simulink model "vehicle_model10DOF_2023b"  (R2023b)
settings: Solver=VariableStepAuto  StartTime=0.0  StopTime=10.0  RelTol=1e-3
values from neighbouring files (symbols this model uses):
  a = 1.05    [model_init.m]
  a0 = 1.6    [pacajeka_init.m]    (also in pacajeka_model_param.mat)
  a1 = -34    [pacajeka_init.m]    (also in pacajeka_model_param.mat)
  a2 = 1250    [pacajeka_init.m]    (also in pacajeka_model_param.mat)
  a3 = 2320    [pacajeka_init.m]    (also in pacajeka_model_param.mat)
  a4 = 12.8    [pacajeka_init.m]    (also in pacajeka_model_param.mat)
  a5 = 0    [pacajeka_init.m]    (also in pacajeka_model_param.mat)
  a6 = -0.0053    [pacajeka_init.m]    (also in pacajeka_model_param.mat)
  a7 = 0.1925    [pacajeka_init.m]    (also in pacajeka_model_param.mat)
  a8 = 0    [pacajeka_init.m]    (also in pacajeka_model_param.mat)
  b = 1.8-a    (= 0.75)    [model_init.m]
  b0 = 1.55    [pacajeka_init.m]    (also in pacajeka_model_param.mat)
  b1 = 0    [pacajeka_init.m]    (also in pacajeka_model_param.mat)
  b2 = 1000    [pacajeka_init.m]    (also in pacajeka_model_param.mat)
  b3 = 60    [pacajeka_init.m]    (also in pacajeka_model_param.mat)
  b4 = 300    [pacajeka_init.m]    (also in pacajeka_model_param.mat)
  b5 = 0.17    [pacajeka_init.m]    (also in pacajeka_model_param.mat)
  b6 = 0    [pacajeka_init.m]    (also in pacajeka_model_param.mat)
  b7 = 0    [pacajeka_init.m]    (also in pacajeka_model_param.mat)
  b8 = 0.2    [pacajeka_init.m]    (also in pacajeka_model_param.mat)
  Bd = 0.1    [model_init.m]
  c = 1.5    [model_init.m]
  I = m*a*b    (= 1496.25)    [model_init.m]
  Idf = 0.805    [model_init.m]
  Idr = 0.805    [model_init.m]
  m = 1900    [model_init.m]
  r = 0.3284    [model_init.m]
  sel_ext = 1    [simulation_init.m]
undefined symbols (not defined in the file or in its folder): Fz_f, Fz_r, mu, sel_int, selector_traj
settings Model: Creator=Ivona  LastModifiedBy=Milosh Yokich
settings SolverCC: AlgebraicLoopSolver=TrustRegion
settings DebuggingCC: UnconnectedInputMsg=warning  UnconnectedOutputMsg=warning  UnconnectedLineMsg=warning
settings ModelReferenceCC: EnableRefExpFcnMdlSchedulingChecks=on

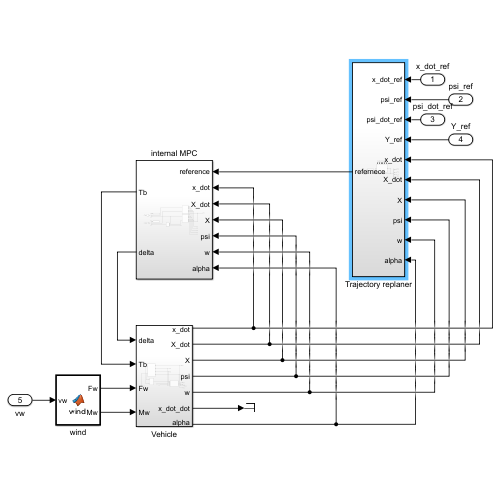
[thumbnail: Simulink's stored preview of the top-level diagram]
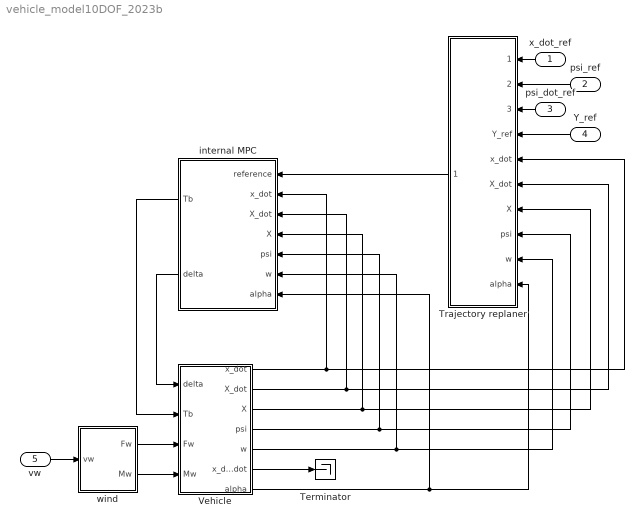
== system vehicle_model10DOF_2023b ==
  x_dot_ref : Inport
  psi_ref : Inport  Port=2
  psi_dot_ref : Inport  Port=3
  Y_ref : Inport  Port=4
  vw : Inport  Port=5
  Terminator : Terminator
  Trajectory replaner : Subsystem
  Vehicle : Subsystem
  internal MPC : Subsystem
  wind : MATLAB Function  TreatAsAtomicUnit=on
  wires:
  vw/1 -> wind/1(vw)
  wind/1(Fw) -> Vehicle/3(Fw)
  wind/2(Mw) -> Vehicle/4(Mw)
  Y_ref/1 -> Trajectory replaner/4(Y_ref)
  x_dot_ref/1 -> Trajectory replaner/1(x_dot_ref)
  Trajectory replaner/1(refernece) -> internal MPC/1(reference)
  Vehicle/1(x_dot) -> Trajectory replaner/5(x_dot), internal MPC/2(x_dot)
  Vehicle/2(X_dot) -> Trajectory replaner/6(X_dot), internal MPC/3(X_dot)
  Vehicle/3(X) -> Trajectory replaner/7(X), internal MPC/4(X)
  Vehicle/4(psi) -> internal MPC/5(psi), Trajectory replaner/8(psi)
  Vehicle/5(w) -> Trajectory replaner/9(w), internal MPC/6(w)
  Vehicle/7(alpha) -> internal MPC/7(alpha), Trajectory replaner/10(alpha)
  internal MPC/2(delta) -> Vehicle/1(delta)
  internal MPC/1(Tb) -> Vehicle/2(Tb)
  psi_ref/1 -> Trajectory replaner/2(psi_ref)
  psi_dot_ref/1 -> Trajectory replaner/3(psi_dot_ref)
  Vehicle/6(x_dot_dot) -> Terminator/1

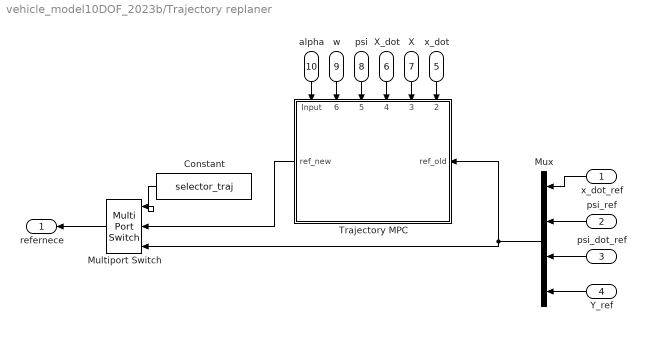
== system vehicle_model10DOF_2023b/Trajectory replaner ==
  x_dot_ref : Inport
  psi_ref : Inport  Port=2
  psi_dot_ref : Inport  Port=3
  Y_ref : Inport  Port=4
  x_dot : Inport  Port=5
  X_dot : Inport  Port=6
  X : Inport  Port=7
  psi : Inport  Port=8
  w : Inport  Port=9
  alpha : Inport  Port=10
  Constant : Constant  Value=selector_traj
  Multiport Switch : MultiPortSwitch  Inputs=2  SaturateOnIntegerOverflow=off  InputSameDT=off
  Mux : Mux
  Trajectory MPC : Subsystem
      settings: PortSchema="{\"entries\":[{\"content\":{\"sides\":[{\"content\":{\"connectorIds\":[\"In1\"]},\"type\":\"ConnectorPlacement.EquallySpacedRectSide\",\"uuid\":\"5ec2c832-fa9f-493b-8380-016dd887c842\"},{\"content\":{\"connectorIds\":[\"Out1\"],\"side\":\"RIGHT\"},\"type\":\"ConnectorPlacement.EquallySpacedRectSide\",\"uuid\":\"21ee5341-71c7-4b30-8141-5e8e6df31cb2\"},{\"content\":{\"connectorIds\":[\"In2\",\"In3\",\"In4\",\"In5\",\"In6\",\"In7\"],\"side\":\"TOP\"},\"type\":\"ConnectorPlacement.EquallySpacedRectSide\",\"uuid\":\"2a2e668d-b31a-4bfa-bdaa-b7e6028e693e\"}]},\"type\":\"ConnectorPlacement.EquallySpacedConnector\",\"uuid\":\"a4f0b61b-50b5-4214-8501-a2ac3a38ae34\"}],\"packageUris\":[\"http://schema.mathworks.com/mf0/Connector/R2020b\"],\"version\":\"1.0\"}"
  refernece : Outport
  wires:
  x_dot_ref/1 -> Mux/1
  psi_ref/1 -> Mux/2
  psi_dot_ref/1 -> Mux/3
  Y_ref/1 -> Mux/4
  Multiport Switch/1 -> refernece/1
  Constant/1 -> Multiport Switch/1
  Mux/1 -> Multiport Switch/3, Trajectory MPC/1(ref_old)
  Trajectory MPC/1(ref_new) -> Multiport Switch/2
  alpha/1 -> Trajectory MPC/7(Input)
  w/1 -> Trajectory MPC/6(Input1)
  psi/1 -> Trajectory MPC/5(Input2)
  x_dot/1 -> Trajectory MPC/2(Input5)
  X_dot/1 -> Trajectory MPC/4(Input3)
  X/1 -> Trajectory MPC/3(Input4)

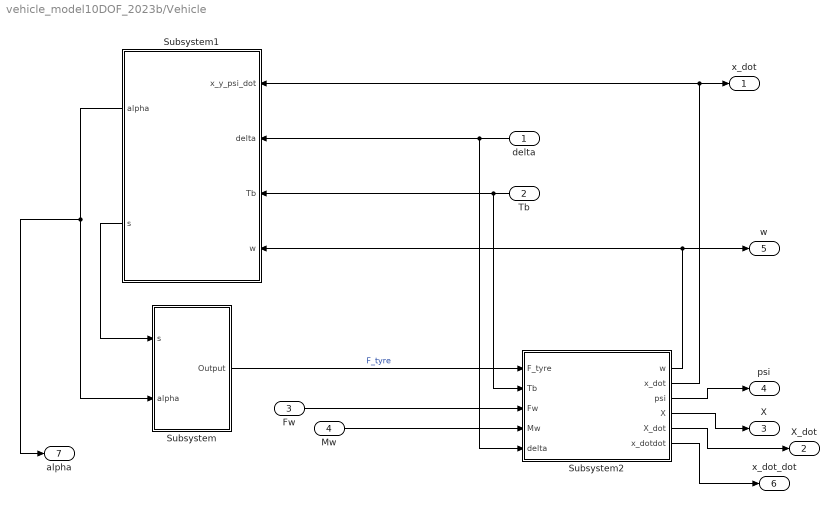
== system vehicle_model10DOF_2023b/Vehicle ==
  delta : Inport
  Tb : Inport  Port=2
  Fw : Inport  Port=3
  Mw : Inport  Port=4
  Subsystem : Subsystem
  Subsystem1 : Subsystem
  Subsystem2 : Subsystem
  x_dot : Outport
  X_dot : Outport  Port=2
  X : Outport  Port=3
  psi : Outport  Port=4
  w : Outport  Port=5
  x_dot_dot : Outport  Port=6
  alpha : Outport  Port=7
  wires:
  Subsystem2/5(X_dot) -> X_dot/1
  Subsystem2/2(x_dot) -> Subsystem1/1(x_y_psi_dot), x_dot/1
  Subsystem/1(Output) -> Subsystem2/1(F_tyre)  "F_tyre"
  Tb/1 -> Subsystem2/2(Tb), Subsystem1/3(Tb)
  Subsystem2/1(w) -> w/1, Subsystem1/4(w)
  Subsystem1/1(alpha) -> alpha/1, Subsystem/2(alpha)
  Subsystem1/2(s) -> Subsystem/1(s)
  Fw/1 -> Subsystem2/3(Fw)
  delta/1 -> Subsystem2/5(delta), Subsystem1/2(delta)
  Mw/1 -> Subsystem2/4(Mw)
  Subsystem2/4(X) -> X/1
  Subsystem2/3(psi) -> psi/1
  Subsystem2/6(x_dotdot) -> x_dot_dot/1

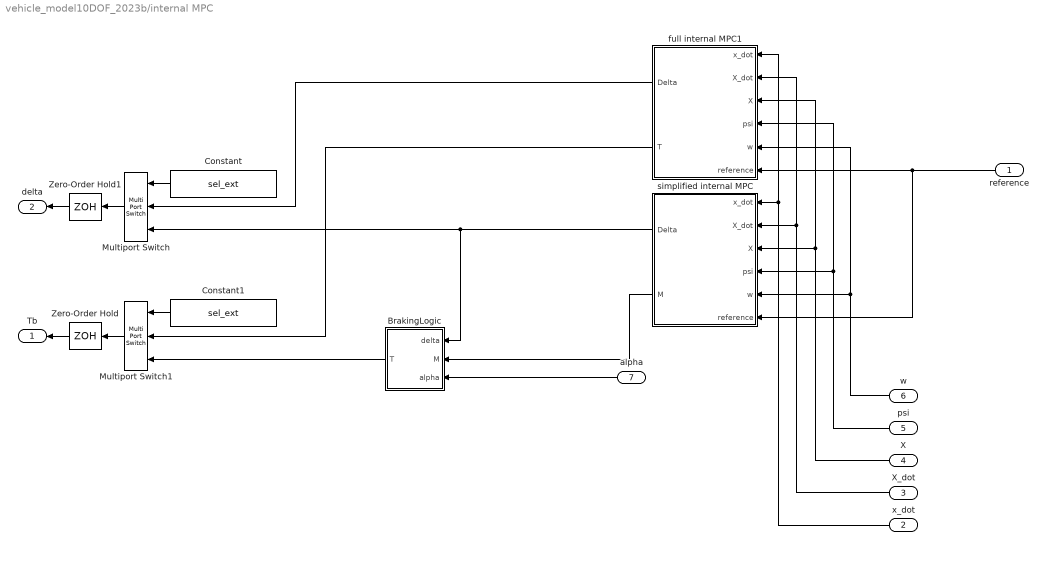
== system vehicle_model10DOF_2023b/internal MPC ==
  reference : Inport
  x_dot : Inport  Port=2
  X_dot : Inport  Port=3
  X : Inport  Port=4
  psi : Inport  Port=5
  w : Inport  Port=6
  alpha : Inport  Port=7
  BrakingLogic : Subsystem
  Constant : Constant  Value=sel_ext
  Constant1 : Constant  Value=sel_ext
  Multiport Switch : MultiPortSwitch  Inputs=2  SaturateOnIntegerOverflow=off  InputSameDT=off
  Multiport Switch1 : MultiPortSwitch  Inputs=2  SaturateOnIntegerOverflow=off  InputSameDT=off
  Zero-Order Hold : ZeroOrderHold  SampleTime=-1
  Zero-Order Hold1 : ZeroOrderHold  SampleTime=-1
  full internal MPC1 : Subsystem
  simplified internal MPC : Subsystem
  Tb : Outport
  delta : Outport  Port=2
  wires:
  simplified internal MPC/1(Delta) -> Multiport Switch/3, BrakingLogic/1(delta)
  X_dot/1 -> full internal MPC1/2(X_dot), simplified internal MPC/2(X_dot)
  Constant/1 -> Multiport Switch/1
  reference/1 -> simplified internal MPC/6(reference), full internal MPC1/6(reference)
  full internal MPC1/2(T) -> Multiport Switch1/2
  Multiport Switch/1 -> Zero-Order Hold1/1
  x_dot/1 -> full internal MPC1/1(x_dot), simplified internal MPC/1(x_dot)
  alpha/1 -> BrakingLogic/3(alpha)
  BrakingLogic/1(T) -> Multiport Switch1/3
  simplified internal MPC/2(M) -> BrakingLogic/2(M)
  psi/1 -> full internal MPC1/4(psi), simplified internal MPC/4(psi)
  Constant1/1 -> Multiport Switch1/1
  full internal MPC1/1(Delta) -> Multiport Switch/2
  Multiport Switch1/1 -> Zero-Order Hold/1
  X/1 -> full internal MPC1/3(X), simplified internal MPC/3(X)
  w/1 -> full internal MPC1/5(w), simplified internal MPC/5(w)
  Zero-Order Hold/1 -> Tb/1
  Zero-Order Hold1/1 -> delta/1

== system vehicle_model10DOF_2023b/Trajectory replaner/Trajectory MPC ==
  ref_old : Inport
  Input5 : Inport  Port=2
  Input4 : Inport  Port=3
  Input3 : Inport  Port=4
  Input2 : Inport  Port=5
  Input1 : Inport  Port=6
  Input : Inport  Port=7
  MATLAB Function : MATLAB Function  TreatAsAtomicUnit=on
  ref_new : Outport
  wires:
  ref_old/1 -> MATLAB Function/1(u)
  MATLAB Function/1(y) -> ref_new/1

== system vehicle_model10DOF_2023b/Vehicle/Subsystem ==
  s : Inport
  alpha : Inport  Port=2
  Demux : Demux
  Demux1 : Demux
  Mux : Mux  Inputs=8
  Subsystem4 : Subsystem
  Output : Outport
  wires:
  Subsystem4/2(Fyfl) -> Mux/2
  Subsystem4/8(Fyfl3) -> Mux/8
  Demux/4 -> Subsystem4/4(Input6)
  Subsystem4/5(Fxfl2) -> Mux/5
  Subsystem4/7(Fxfl3) -> Mux/7
  alpha/1 -> Demux1/1
  Demux/1 -> Subsystem4/1(Input)
  Subsystem4/3(Fxfl1) -> Mux/3
  Subsystem4/4(Fyfl1) -> Mux/4
  Demux/2 -> Subsystem4/2(Input2)
  Subsystem4/6(Fyfl2) -> Mux/6
  Demux/3 -> Subsystem4/3(Input4)
  Subsystem4/1(Fxfl) -> Mux/1
  Demux1/1 -> Subsystem4/5(Input1)
  Demux1/2 -> Subsystem4/6(Input3)
  Demux1/4 -> Subsystem4/8(Input7)
  Demux1/3 -> Subsystem4/7(Input5)
  s/1 -> Demux/1
  Mux/1 -> Output/1  "F"

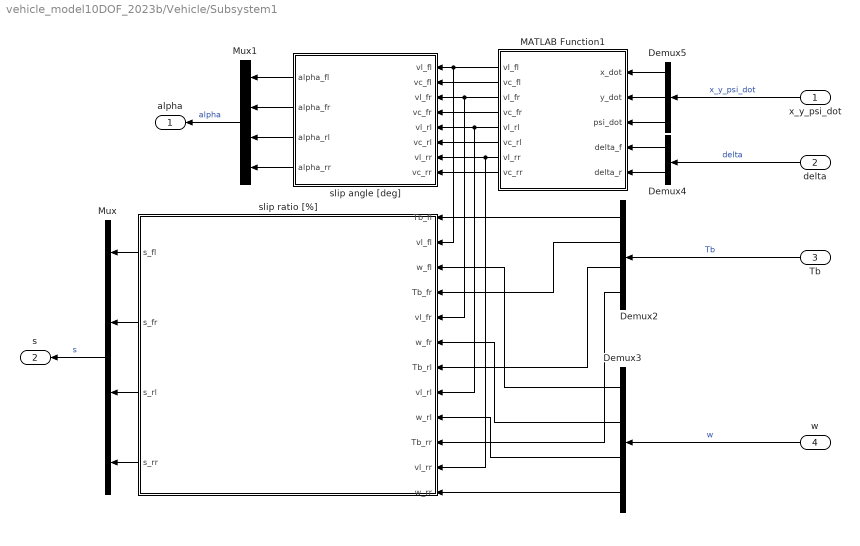
== system vehicle_model10DOF_2023b/Vehicle/Subsystem1 ==
  x_y_psi_dot : Inport
  delta : Inport  Port=2
  Tb : Inport  Port=3
  w : Inport  Port=4
  Demux2 : Demux
  Demux3 : Demux
  Demux4 : Demux  Outputs=2
  Demux5 : Demux  Outputs=3
  MATLAB Function1 : MATLAB Function  TreatAsAtomicUnit=on
  Mux : Mux
  Mux1 : Mux
  slip angle [deg] : MATLAB Function  TreatAsAtomicUnit=on
  slip ratio [%] : Subsystem
  alpha : Outport
  s : Outport  Port=2
  wires:
  Demux4/1 -> MATLAB Function1/4(delta_f)
  slip ratio [%]/3(s_rl) -> Mux/3
  Mux1/1 -> alpha/1  "alpha"
  MATLAB Function1/5(vl_rl) -> slip ratio [%]/8(vl_rl), slip angle [deg]/5(vl_rl)
  Demux2/1 -> slip ratio [%]/1(Tb_fl)
  slip ratio [%]/1(s_fl) -> Mux/1
  MATLAB Function1/7(vl_rr) -> slip ratio [%]/11(vl_rr), slip angle [deg]/7(vl_rr)
  slip ratio [%]/4(s_rr) -> Mux/4
  delta/1 -> Demux4/1  "delta"
  Demux5/3 -> MATLAB Function1/3(psi_dot)
  MATLAB Function1/3(vl_fr) -> slip ratio [%]/5(vl_fr), slip angle [deg]/3(vl_fr)
  slip angle [deg]/3(alpha_rl) -> Mux1/3
  MATLAB Function1/1(vl_fl) -> slip ratio [%]/2(vl_fl), slip angle [deg]/1(vl_fl)
  slip angle [deg]/4(alpha_rr) -> Mux1/4
  MATLAB Function1/8(vc_rr) -> slip angle [deg]/8(vc_rr)
  Demux3/1 -> slip ratio [%]/3(w_fl)
  slip ratio [%]/2(s_fr) -> Mux/2
  Demux5/1 -> MATLAB Function1/1(x_dot)
  MATLAB Function1/2(vc_fl) -> slip angle [deg]/2(vc_fl)
  x_y_psi_dot/1 -> Demux5/1  "x_y_psi_dot"
  slip angle [deg]/1(alpha_fl) -> Mux1/1
  w/1 -> Demux3/1  "w"
  MATLAB Function1/4(vc_fr) -> slip angle [deg]/4(vc_fr)
  slip angle [deg]/2(alpha_fr) -> Mux1/2
  Demux5/2 -> MATLAB Function1/2(y_dot)
  MATLAB Function1/6(vc_rl) -> slip angle [deg]/6(vc_rl)
  Demux2/2 -> slip ratio [%]/4(Tb_fr)
  Demux3/2 -> slip ratio [%]/6(w_fr)
  Demux3/4 -> slip ratio [%]/12(w_rr)
  Demux2/3 -> slip ratio [%]/7(Tb_rl)
  Demux2/4 -> slip ratio [%]/10(Tb_rr)
  Demux4/2 -> MATLAB Function1/5(delta_r)
  Demux3/3 -> slip ratio [%]/9(w_rl)
  Tb/1 -> Demux2/1  "Tb"
  Mux/1 -> s/1  "s"

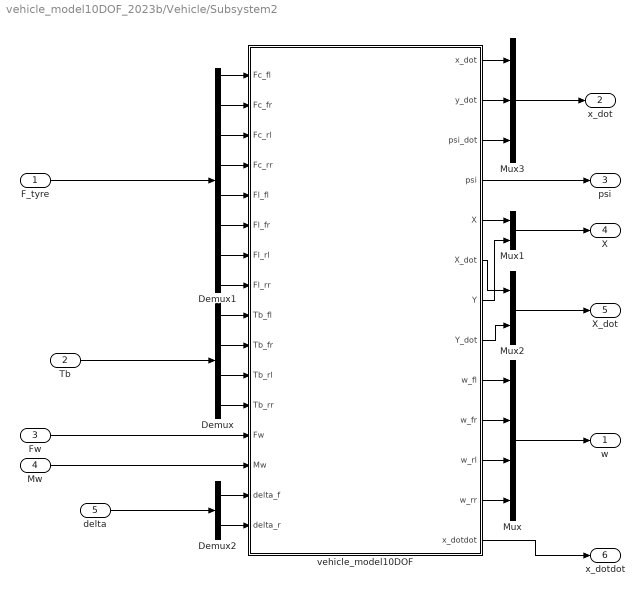
== system vehicle_model10DOF_2023b/Vehicle/Subsystem2 ==
  F_tyre : Inport
  Tb : Inport  Port=2
  Fw : Inport  Port=3
  Mw : Inport  Port=4
  delta : Inport  Port=5
  Demux : Demux
  Demux1 : Demux  Outputs=8
  Demux2 : Demux  Outputs=2
  Mux : Mux
  Mux1 : Mux  Inputs=2
  Mux2 : Mux  Inputs=2
  Mux3 : Mux  Inputs=3
  vehicle_model10DOF : Subsystem
  w : Outport
  x_dot : Outport  Port=2
  psi : Outport  Port=3
  X : Outport  Port=4
  X_dot : Outport  Port=5
  x_dotdot : Outport  Port=6
  wires:
  Demux1/6 -> vehicle_model10DOF/6(Fl_fr)
  vehicle_model10DOF/3(psi_dot) -> Mux3/3
  Mux3/1 -> x_dot/1
  Demux2/2 -> vehicle_model10DOF/16(delta_r)
  Mux2/1 -> X_dot/1
  vehicle_model10DOF/2(y_dot) -> Mux3/2
  vehicle_model10DOF/12(w_rr) -> Mux/4
  Demux1/8 -> vehicle_model10DOF/8(Fl_rr)
  vehicle_model10DOF/8(Y_dot) -> Mux2/2
  vehicle_model10DOF/1(x_dot) -> Mux3/1
  Demux/3 -> vehicle_model10DOF/11(Tb_rl)
  vehicle_model10DOF/9(w_fl) -> Mux/1
  Demux/2 -> vehicle_model10DOF/10(Tb_fr)
  Demux1/7 -> vehicle_model10DOF/7(Fl_rl)
  Demux1/5 -> vehicle_model10DOF/5(Fl_fl)
  Mux/1 -> w/1
  Demux/4 -> vehicle_model10DOF/12(Tb_rr)
  Demux1/3 -> vehicle_model10DOF/3(Fc_rl)
  Demux1/4 -> vehicle_model10DOF/4(Fc_rr)
  Demux/1 -> vehicle_model10DOF/9(Tb_fl)
  Demux1/2 -> vehicle_model10DOF/2(Fc_fr)
  Demux1/1 -> vehicle_model10DOF/1(Fc_fl)
  vehicle_model10DOF/7(Y) -> Mux1/2
  vehicle_model10DOF/10(w_fr) -> Mux/2
  Demux2/1 -> vehicle_model10DOF/15(delta_f)
  vehicle_model10DOF/5(X) -> Mux1/1
  vehicle_model10DOF/11(w_rl) -> Mux/3
  Fw/1 -> vehicle_model10DOF/13(Fw)
  vehicle_model10DOF/6(X_dot) -> Mux2/1
  Mw/1 -> vehicle_model10DOF/14(Mw)
  F_tyre/1 -> Demux1/1
  Tb/1 -> Demux/1
  vehicle_model10DOF/4(psi) -> psi/1
  Mux1/1 -> X/1
  delta/1 -> Demux2/1
  vehicle_model10DOF/13(x_dotdot) -> x_dotdot/1

== system vehicle_model10DOF_2023b/internal MPC/BrakingLogic ==
  delta : Inport
  M : Inport  Port=2
  alpha : Inport  Port=3
  Demux : Demux
  MATLAB Function : MATLAB Function  TreatAsAtomicUnit=on
  MATLAB Function1 : MATLAB Function  TreatAsAtomicUnit=on
  Mux : Mux
  T : Outport
  wires:
  MATLAB Function/4(Tbrr) -> Mux/4
  Demux/1 -> MATLAB Function1/1(alpha_fl)
  MATLAB Function/3(Tbrl) -> Mux/3
  MATLAB Function/2(Tbfr) -> Mux/2
  M/1 -> MATLAB Function/4(M)
  Demux/4 -> MATLAB Function1/4(alpha_rr)
  MATLAB Function/1(Tbfl) -> Mux/1
  Demux/3 -> MATLAB Function1/3(alpha_rl)
  MATLAB Function1/1(alpha_f) -> MATLAB Function/2(alpha_f)
  alpha/1 -> Demux/1
  Demux/2 -> MATLAB Function1/2(alpha_fr)
  MATLAB Function1/2(alpha_r) -> MATLAB Function/3(alpha_r)
  Mux/1 -> T/1
  delta/1 -> MATLAB Function/1(delta)

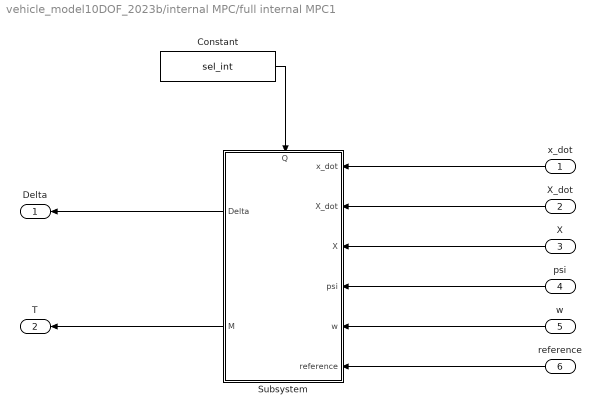
== system vehicle_model10DOF_2023b/internal MPC/full internal MPC1 ==
  x_dot : Inport
  X_dot : Inport  Port=2
  X : Inport  Port=3
  psi : Inport  Port=4
  w : Inport  Port=5
  reference : Inport  Port=6
  Constant : Constant  Value=sel_int
  Subsystem : Subsystem
      settings: PortSchema="{\"entries\":[{\"content\":{\"sides\":[{\"content\":{\"connectorIds\":[\"In1\",\"In2\",\"In3\",\"In4\",\"In5\",\"In6\"]},\"type\":\"ConnectorPlacement.EquallySpacedRectSide\",\"uuid\":\"afc2eced-fac6-40c0-835b-934651f4342e\"},{\"content\":{\"connectorIds\":[\"Out1\",\"Out2\"],\"side\":\"RIGHT\"},\"type\":\"ConnectorPlacement.EquallySpacedRectSide\",\"uuid\":\"0398ea9e-d615-4012-a81d-0e7d9c0762e8\"},{\"content\":{\"connectorIds\":[\"In7\"],\"side\":\"TOP\"},\"type\":\"ConnectorPlacement.EquallySpacedRectSide\",\"uuid\":\"ccaf2262-c403-4668-80a8-85ac531d9aa6\"}]},\"type\":\"ConnectorPlacement.EquallySpacedConnector\",\"uuid\":\"6d745792-8d70-46c2-89f7-22992c5da21d\"}],\"packageUris\":[\"http://schema.mathworks.com/mf0/Connector/R2020b\"],\"version\":\"1.0\"}"
  Delta : Outport
  T : Outport  Port=2
  wires:
  x_dot/1 -> Subsystem/1(x_dot)
  X_dot/1 -> Subsystem/2(X_dot)
  X/1 -> Subsystem/3(X)
  psi/1 -> Subsystem/4(psi)
  w/1 -> Subsystem/5(w)
  reference/1 -> Subsystem/6(reference)
  Constant/1 -> Subsystem/7(Q)
  Subsystem/1(Delta) -> Delta/1
  Subsystem/2(M) -> T/1

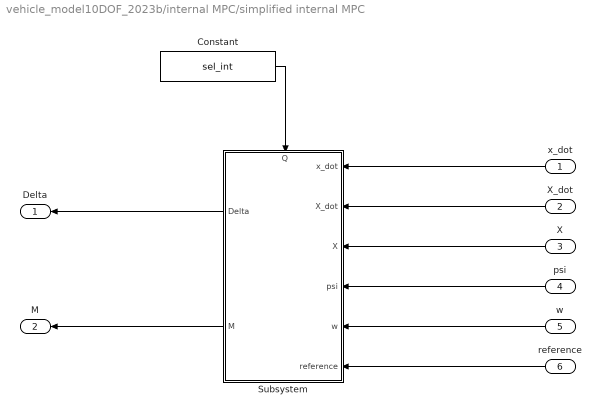
== system vehicle_model10DOF_2023b/internal MPC/simplified internal MPC ==
  x_dot : Inport
  X_dot : Inport  Port=2
  X : Inport  Port=3
  psi : Inport  Port=4
  w : Inport  Port=5
  reference : Inport  Port=6
  Constant : Constant  Value=sel_int
  Subsystem : Subsystem
      settings: PortSchema="{\"entries\":[{\"content\":{\"sides\":[{\"content\":{\"connectorIds\":[\"In1\",\"In2\",\"In3\",\"In4\",\"In5\",\"In6\"]},\"type\":\"ConnectorPlacement.EquallySpacedRectSide\",\"uuid\":\"afc2eced-fac6-40c0-835b-934651f4342e\"},{\"content\":{\"connectorIds\":[\"Out1\",\"Out2\"],\"side\":\"RIGHT\"},\"type\":\"ConnectorPlacement.EquallySpacedRectSide\",\"uuid\":\"0398ea9e-d615-4012-a81d-0e7d9c0762e8\"},{\"content\":{\"connectorIds\":[\"In7\"],\"side\":\"TOP\"},\"type\":\"ConnectorPlacement.EquallySpacedRectSide\",\"uuid\":\"ccaf2262-c403-4668-80a8-85ac531d9aa6\"}]},\"type\":\"ConnectorPlacement.EquallySpacedConnector\",\"uuid\":\"6d745792-8d70-46c2-89f7-22992c5da21d\"}],\"packageUris\":[\"http://schema.mathworks.com/mf0/Connector/R2020b\"],\"version\":\"1.0\"}"
  Delta : Outport
  M : Outport  Port=2
  wires:
  x_dot/1 -> Subsystem/1(x_dot)
  X_dot/1 -> Subsystem/2(X_dot)
  X/1 -> Subsystem/3(X)
  psi/1 -> Subsystem/4(psi)
  w/1 -> Subsystem/5(w)
  reference/1 -> Subsystem/6(reference)
  Constant/1 -> Subsystem/7(Q)
  Subsystem/1(Delta) -> Delta/1
  Subsystem/2(M) -> M/1

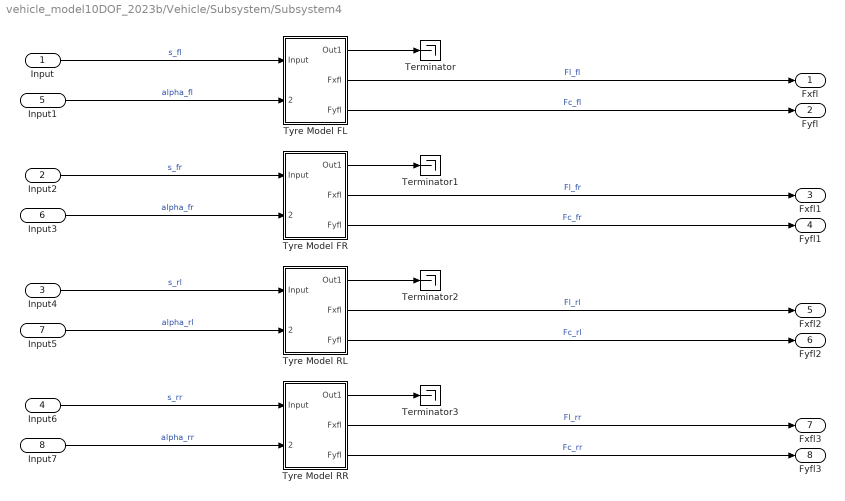
== system vehicle_model10DOF_2023b/Vehicle/Subsystem/Subsystem4 ==
  Input : Inport
  Input2 : Inport  Port=2
  Input4 : Inport  Port=3
  Input6 : Inport  Port=4
  Input1 : Inport  Port=5
  Input3 : Inport  Port=6
  Input5 : Inport  Port=7
  Input7 : Inport  Port=8
  Terminator{,1..3} (4 alike) : Terminator
  Tyre Model FL : Subsystem
  Tyre Model FR : Subsystem
  Tyre Model RL : Subsystem
  Tyre Model RR : Subsystem
  Fxfl : Outport
  Fyfl : Outport  Port=2
  Fxfl1 : Outport  Port=3
  Fyfl1 : Outport  Port=4
  Fxfl2 : Outport  Port=5
  Fyfl2 : Outport  Port=6
  Fxfl3 : Outport  Port=7
  Fyfl3 : Outport  Port=8
  wires:
  Input/1 -> Tyre Model FL/1(Input)  "s_fl"
  Input1/1 -> Tyre Model FL/2(Input1)  "alpha_fl"
  Tyre Model FL/1(Out1) -> Terminator/1
  Tyre Model FL/3(Fyfl) -> Fyfl/1  "Fc_fl"
  Tyre Model FL/2(Fxfl) -> Fxfl/1  "Fl_fl"
  Input2/1 -> Tyre Model FR/1(Input)  "s_fr"
  Input3/1 -> Tyre Model FR/2(Input1)  "alpha_fr"
  Tyre Model FR/2(Fxfl) -> Fxfl1/1  "Fl_fr"
  Tyre Model FR/1(Out1) -> Terminator1/1
  Tyre Model FR/3(Fyfl) -> Fyfl1/1  "Fc_fr"
  Input4/1 -> Tyre Model RL/1(Input)  "s_rl"
  Input5/1 -> Tyre Model RL/2(Input1)  "alpha_rl"
  Tyre Model RL/2(Fxfl) -> Fxfl2/1  "Fl_rl"
  Tyre Model RL/1(Out1) -> Terminator2/1
  Tyre Model RL/3(Fyfl) -> Fyfl2/1  "Fc_rl"
  Input6/1 -> Tyre Model RR/1(Input)  "s_rr"
  Input7/1 -> Tyre Model RR/2(Input1)  "alpha_rr"
  Tyre Model RR/2(Fxfl) -> Fxfl3/1  "Fl_rr"
  Tyre Model RR/1(Out1) -> Terminator3/1
  Tyre Model RR/3(Fyfl) -> Fyfl3/1  "Fc_rr"

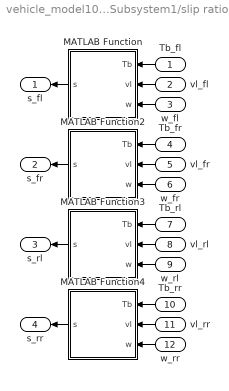
== system vehicle_model10DOF_2023b/Vehicle/Subsystem1/slip ratio [%] ==
  Tb_fl : Inport
  vl_fl : Inport  Port=2
  w_fl : Inport  Port=3
  Tb_fr : Inport  Port=4
  vl_fr : Inport  Port=5
  w_fr : Inport  Port=6
  Tb_rl : Inport  Port=7
  vl_rl : Inport  Port=8
  w_rl : Inport  Port=9
  Tb_rr : Inport  Port=10
  vl_rr : Inport  Port=11
  w_rr : Inport  Port=12
  MATLAB Function : MATLAB Function  TreatAsAtomicUnit=on
  MATLAB Function2 : MATLAB Function  TreatAsAtomicUnit=on
  MATLAB Function3 : MATLAB Function  TreatAsAtomicUnit=on
  MATLAB Function4 : MATLAB Function  TreatAsAtomicUnit=on
  s_fl : Outport
  s_fr : Outport  Port=2
  s_rl : Outport  Port=3
  s_rr : Outport  Port=4
  wires:
  vl_rl/1 -> MATLAB Function3/2(vl)
  Tb_rl/1 -> MATLAB Function3/1(Tb)
  w_rl/1 -> MATLAB Function3/3(w)
  vl_rr/1 -> MATLAB Function4/2(vl)
  MATLAB Function2/1(s) -> s_fr/1
  MATLAB Function3/1(s) -> s_rl/1
  Tb_fl/1 -> MATLAB Function/1(Tb)
  w_fr/1 -> MATLAB Function2/3(w)
  Tb_fr/1 -> MATLAB Function2/1(Tb)
  w_rr/1 -> MATLAB Function4/3(w)
  MATLAB Function4/1(s) -> s_rr/1
  vl_fl/1 -> MATLAB Function/2(vl)
  w_fl/1 -> MATLAB Function/3(w)
  vl_fr/1 -> MATLAB Function2/2(vl)
  MATLAB Function/1(s) -> s_fl/1
  Tb_rr/1 -> MATLAB Function4/1(Tb)

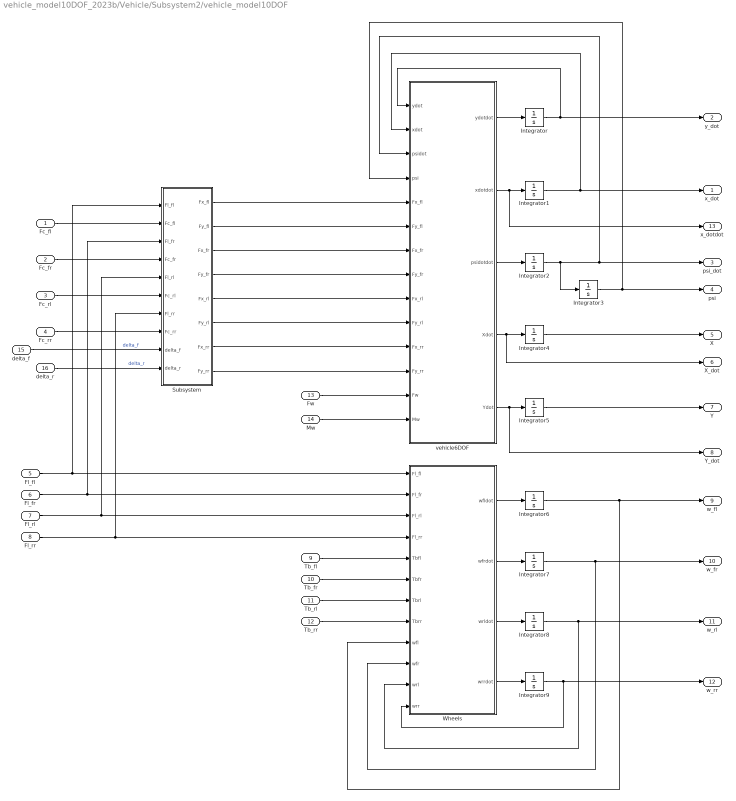
== system vehicle_model10DOF_2023b/Vehicle/Subsystem2/vehicle_model10DOF ==
  Fc_fl : Inport
  Fc_fr : Inport  Port=2
  Fc_rl : Inport  Port=3
  Fc_rr : Inport  Port=4
  Fl_fl : Inport  Port=5
  Fl_fr : Inport  Port=6
  Fl_rl : Inport  Port=7
  Fl_rr : Inport  Port=8
  Tb_fl : Inport  Port=9
  Tb_fr : Inport  Port=10
  Tb_rl : Inport  Port=11
  Tb_rr : Inport  Port=12
  Fw : Inport  Port=13
  Mw : Inport  Port=14
  delta_f : Inport  Port=15
  delta_r : Inport  Port=16
  Integrator{,1..9} (10 alike) : Integrator
  Subsystem : Subsystem
  Wheels : MATLAB Function  TreatAsAtomicUnit=on
  vehicle6DOF : MATLAB Function  TreatAsAtomicUnit=on
  x_dot : Outport
  y_dot : Outport  Port=2
  psi_dot : Outport  Port=3
  psi : Outport  Port=4
  X : Outport  Port=5
  X_dot : Outport  Port=6
  Y : Outport  Port=7
  Y_dot : Outport  Port=8
  w_fl : Outport  Port=9
  w_fr : Outport  Port=10
  w_rl : Outport  Port=11
  w_rr : Outport  Port=12
  x_dotdot : Outport  Port=13
  wires:
  vehicle6DOF/1(ydotdot) -> Integrator/1
  Integrator/1 -> y_dot/1, vehicle6DOF/1(ydot)
  vehicle6DOF/2(xdotdot) -> x_dotdot/1, Integrator1/1
  Integrator1/1 -> x_dot/1, vehicle6DOF/2(xdot)
  vehicle6DOF/3(psidotdot) -> Integrator2/1
  Integrator2/1 -> Integrator3/1, vehicle6DOF/3(psidot), psi_dot/1
  Integrator3/1 -> psi/1, vehicle6DOF/4(psi)
  Integrator4/1 -> X/1
  vehicle6DOF/4(Xdot) -> X_dot/1, Integrator4/1
  vehicle6DOF/5(Ydot) -> Y_dot/1, Integrator5/1
  Integrator5/1 -> Y/1
  Fw/1 -> vehicle6DOF/13(Fw)
  Mw/1 -> vehicle6DOF/14(Mw)
  Wheels/1(wfldot) -> Integrator6/1
  Wheels/2(wfrdot) -> Integrator7/1
  Wheels/3(wrldot) -> Integrator8/1
  Wheels/4(wrrdot) -> Integrator9/1
  Integrator6/1 -> w_fl/1, Wheels/9(wfl)
  Integrator7/1 -> Wheels/10(wfr), w_fr/1
  Integrator9/1 -> Wheels/12(wrr), w_rr/1
  Integrator8/1 -> Wheels/11(wrl), w_rl/1
  Tb_fl/1 -> Wheels/5(Tbfl)
  Tb_fr/1 -> Wheels/6(Tbfr)
  Tb_rl/1 -> Wheels/7(Tbrl)
  Tb_rr/1 -> Wheels/8(Tbrr)
  Fl_fl/1 -> Subsystem/1(Fl_fl), Wheels/1(Fl_fl)
  Fl_fr/1 -> Subsystem/3(Fl_fr), Wheels/2(Fl_fr)
  Fl_rl/1 -> Wheels/3(Fl_rl), Subsystem/5(Fl_rl)
  Fl_rr/1 -> Wheels/4(Fl_rr), Subsystem/7(Fl_rr)
  Subsystem/1(Fx_fl) -> vehicle6DOF/5(Fx_fl)
  Subsystem/2(Fy_fl) -> vehicle6DOF/6(Fy_fl)
  Subsystem/3(Fx_fr) -> vehicle6DOF/7(Fx_fr)
  Subsystem/4(Fy_fr) -> vehicle6DOF/8(Fy_fr)
  Subsystem/5(Fx_rl) -> vehicle6DOF/9(Fx_rl)
  Subsystem/6(Fy_rl) -> vehicle6DOF/10(Fy_rl)
  Subsystem/7(Fx_rr) -> vehicle6DOF/11(Fx_rr)
  Subsystem/8(Fy_rr) -> vehicle6DOF/12(Fy_rr)
  delta_f/1 -> Subsystem/9(delta_f)  "delta_f"
  delta_r/1 -> Subsystem/10(delta_r)  "delta_r"
  Fc_rr/1 -> Subsystem/8(Fc_rr)
  Fc_rl/1 -> Subsystem/6(Fc_rl)
  Fc_fr/1 -> Subsystem/4(Fc_fr)
  Fc_fl/1 -> Subsystem/2(Fc_fl)

== system vehicle_model10DOF_2023b/internal MPC/full internal MPC1/Subsystem ==
  x_dot : Inport
  X_dot : Inport  Port=2
  X : Inport  Port=3
  psi : Inport  Port=4
  w : Inport  Port=5
  reference : Inport  Port=6
  Q : Inport  Port=7
  MATLAB Function : MATLAB Function  TreatAsAtomicUnit=on
  Delta : Outport
  M : Outport  Port=2
  wires:
  Q/1 -> MATLAB Function/1(Q)
  MATLAB Function/1(M) -> Delta/1
  MATLAB Function/2(Delta) -> M/1

== system vehicle_model10DOF_2023b/internal MPC/simplified internal MPC/Subsystem ==
  x_dot : Inport
  X_dot : Inport  Port=2
  X : Inport  Port=3
  psi : Inport  Port=4
  w : Inport  Port=5
  reference : Inport  Port=6
  Q : Inport  Port=7
  MATLAB Function : MATLAB Function  TreatAsAtomicUnit=on
  Delta : Outport
  M : Outport  Port=2
  wires:
  Q/1 -> MATLAB Function/1(Q)
  MATLAB Function/1(M) -> Delta/1
  MATLAB Function/2(Delta) -> M/1

== system vehicle_model10DOF_2023b/Vehicle/Subsystem/Subsystem4/Tyre Model FL ==
  Input : Inport
  Input1 : Inport  Port=2
  Combined force : MATLAB Function  TreatAsAtomicUnit=on
  Constant5 : Constant  Value=0
  Constant6 : Constant  Value=0
  "brake force " : MATLAB Function  TreatAsAtomicUnit=on
  side force : MATLAB Function  TreatAsAtomicUnit=on
  Out1 : Outport
  Fxfl : Outport  Port=2
  Fyfl : Outport  Port=3
  wires:
  Input/1 -> Combined force/2(s), "brake force "/1(s)
  Combined force/1(F) -> Out1/1
  Combined force/2(Fx) -> Fxfl/1
  Constant6/1 -> side force/2(Sv)
  Constant5/1 -> side force/3(Sh)
  "brake force "/1(F_x0) -> Combined force/1(F_x0)
  side force/1(F_y0) -> Combined force/3(F_y0)
  Combined force/3(Fy) -> Fyfl/1
  Input1/1 -> Combined force/4(alpha), side force/1(alpha)

== system vehicle_model10DOF_2023b/Vehicle/Subsystem/Subsystem4/Tyre Model FR ==
  Input : Inport
  Input1 : Inport  Port=2
  Combined force : MATLAB Function  TreatAsAtomicUnit=on
  Constant5 : Constant  Value=0
  Constant6 : Constant  Value=0
  "brake force " : MATLAB Function  TreatAsAtomicUnit=on
  side force : MATLAB Function  TreatAsAtomicUnit=on
  Out1 : Outport
  Fxfl : Outport  Port=2
  Fyfl : Outport  Port=3
  wires:
  Input/1 -> Combined force/2(s), "brake force "/1(s)
  Combined force/1(F) -> Out1/1
  Combined force/2(Fx) -> Fxfl/1
  Constant6/1 -> side force/2(Sv)
  Constant5/1 -> side force/3(Sh)
  "brake force "/1(F_x0) -> Combined force/1(F_x0)
  side force/1(F_y0) -> Combined force/3(F_y0)
  Combined force/3(Fy) -> Fyfl/1
  Input1/1 -> Combined force/4(alpha), side force/1(alpha)

== system vehicle_model10DOF_2023b/Vehicle/Subsystem/Subsystem4/Tyre Model RL ==
  Input : Inport
  Input1 : Inport  Port=2
  Combined force : MATLAB Function  TreatAsAtomicUnit=on
  Constant5 : Constant  Value=0
  Constant6 : Constant  Value=0
  "brake force " : MATLAB Function  TreatAsAtomicUnit=on
  side force : MATLAB Function  TreatAsAtomicUnit=on
  Out1 : Outport
  Fxfl : Outport  Port=2
  Fyfl : Outport  Port=3
  wires:
  Input/1 -> Combined force/2(s), "brake force "/1(s)
  Combined force/1(F) -> Out1/1
  Combined force/2(Fx) -> Fxfl/1
  Constant6/1 -> side force/2(Sv)
  Constant5/1 -> side force/3(Sh)
  "brake force "/1(F_x0) -> Combined force/1(F_x0)
  side force/1(F_y0) -> Combined force/3(F_y0)
  Combined force/3(Fy) -> Fyfl/1
  Input1/1 -> Combined force/4(alpha), side force/1(alpha)

== system vehicle_model10DOF_2023b/Vehicle/Subsystem/Subsystem4/Tyre Model RR ==
  Input : Inport
  Input1 : Inport  Port=2
  Combined force : MATLAB Function  TreatAsAtomicUnit=on
  Constant5 : Constant  Value=0
  Constant6 : Constant  Value=0
  "brake force " : MATLAB Function  TreatAsAtomicUnit=on
  side force : MATLAB Function  TreatAsAtomicUnit=on
  Out1 : Outport
  Fxfl : Outport  Port=2
  Fyfl : Outport  Port=3
  wires:
  Input/1 -> Combined force/2(s), "brake force "/1(s)
  Combined force/1(F) -> Out1/1
  Combined force/2(Fx) -> Fxfl/1
  Constant6/1 -> side force/2(Sv)
  Constant5/1 -> side force/3(Sh)
  "brake force "/1(F_x0) -> Combined force/1(F_x0)
  side force/1(F_y0) -> Combined force/3(F_y0)
  Combined force/3(Fy) -> Fyfl/1
  Input1/1 -> Combined force/4(alpha), side force/1(alpha)

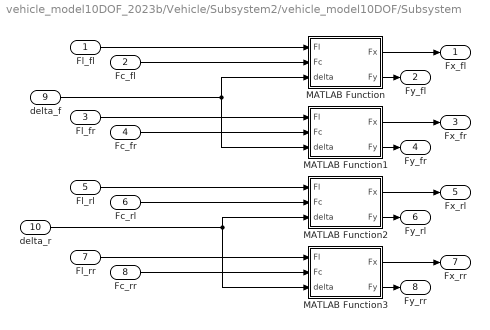
== system vehicle_model10DOF_2023b/Vehicle/Subsystem2/vehicle_model10DOF/Subsystem ==
  Fl_fl : Inport
  Fc_fl : Inport  Port=2
  Fl_fr : Inport  Port=3
  Fc_fr : Inport  Port=4
  Fl_rl : Inport  Port=5
  Fc_rl : Inport  Port=6
  Fl_rr : Inport  Port=7
  Fc_rr : Inport  Port=8
  delta_f : Inport  Port=9
  delta_r : Inport  Port=10
  MATLAB Function : MATLAB Function  TreatAsAtomicUnit=on
  MATLAB Function1 : MATLAB Function  TreatAsAtomicUnit=on
  MATLAB Function2 : MATLAB Function  TreatAsAtomicUnit=on
  MATLAB Function3 : MATLAB Function  TreatAsAtomicUnit=on
  Fx_fl : Outport
  Fy_fl : Outport  Port=2
  Fx_fr : Outport  Port=3
  Fy_fr : Outport  Port=4
  Fx_rl : Outport  Port=5
  Fy_rl : Outport  Port=6
  Fx_rr : Outport  Port=7
  Fy_rr : Outport  Port=8
  wires:
  delta_r/1 -> MATLAB Function2/3(delta), MATLAB Function3/3(delta)
  MATLAB Function2/2(Fy) -> Fy_rl/1
  Fc_fr/1 -> MATLAB Function1/2(Fc)
  MATLAB Function/2(Fy) -> Fy_fl/1
  MATLAB Function/1(Fx) -> Fx_fl/1
  MATLAB Function3/1(Fx) -> Fx_rr/1
  Fl_rl/1 -> MATLAB Function2/1(Fl)
  Fl_rr/1 -> MATLAB Function3/1(Fl)
  Fc_rr/1 -> MATLAB Function3/2(Fc)
  MATLAB Function1/1(Fx) -> Fx_fr/1
  MATLAB Function3/2(Fy) -> Fy_rr/1
  delta_f/1 -> MATLAB Function1/3(delta), MATLAB Function/3(delta)
  Fl_fl/1 -> MATLAB Function/1(Fl)
  Fl_fr/1 -> MATLAB Function1/1(Fl)
  MATLAB Function2/1(Fx) -> Fx_rl/1
  MATLAB Function1/2(Fy) -> Fy_fr/1
  Fc_fl/1 -> MATLAB Function/2(Fc)
  Fc_rl/1 -> MATLAB Function2/2(Fc)

== matlab function vehicle_model10DOF_2023b/Vehicle/Subsystem/Subsystem4/Tyre Model FR/side force ==
  data: alpha input; Sv input; Sh input; F_y0 output; a0 parameter; a1 parameter; a2 parameter; a3 parameter; a4 parameter; a6 parameter; a7 parameter; a5 parameter; a8 parameter; Fz_r parameter; mu parameter
function F_y0 = fcn(alpha, Sv, Sh, a0, a1, a2, a3, a4, a6, ...
    a7, a5, a8, Fz_r, mu)
persistent C D B E

% init persistent variables: 
if isempty(C)
    C = a0;
    D = mu*(a1*Fz_r^2 + a2*Fz_r);
    B = (a3*sin(a4*atan(Fz_r/a5)))/C/D;
    E = a6*Fz_r^2 + a7*Fz_r + a8;

end
X = alpha+Sh;
phi = (1-E)*X + E/B*atan(B*X);
F_y0 = -(D*sin(C*atan(B*phi)) +Sv);

== matlab function vehicle_model10DOF_2023b/Vehicle/Subsystem/Subsystem4/Tyre Model RL/Combined force ==
  data: F_x0 input; F output; s input; F_y0 input; alpha input; Fx output; Fy output
 function [F, Fx, Fy] = fcn(F_x0, s, F_y0, alpha)


% normalization of s
s = s/100;
alpha_rad = alpha/180*pi;

beta = atan2(sin(alpha_rad), s);

Fx = F_x0*abs(cos(beta));

Fy = F_y0*abs(sin(beta));

F =  F_x0*cos(beta)^2 + F_y0*sin(beta)^2;

== matlab function vehicle_model10DOF_2023b/Vehicle/Subsystem/Subsystem4/Tyre Model RL/brake force  ==
  data: s input; F_x0 output; b0 parameter; b1 parameter; b2 parameter; b3 parameter; b4 parameter; b6 parameter; b7 parameter; b5 parameter; b8 parameter; Fz_f parameter; mu parameter
function F_x0 = fcn(s, b0, b1, b2, b3, b4, b6, b7, b5, b8, Fz_f, mu)
persistent C D B E

% init persistent variables: 
if isempty(C)
    C = b0;
    D = mu*(b1*Fz_f^2 + b2*Fz_f);
    B = (b3*Fz_f^2 + b4*Fz_f)/(C*D)*exp(-b5*Fz_f);
    E = b6*Fz_f^2 + b7*Fz_f + b8;

end
X = s;
phi = (1-E)*X + E/B*atan(B*X);
F_x0 = (D*sin(C*atan(B*phi)));

== matlab function vehicle_model10DOF_2023b/Vehicle/Subsystem/Subsystem4/Tyre Model RL/side force ==
  data: alpha input; Sv input; Sh input; F_y0 output; a0 parameter; a1 parameter; a2 parameter; a3 parameter; a4 parameter; a6 parameter; a7 parameter; a5 parameter; a8 parameter; Fz_r parameter; mu parameter
function F_y0 = fcn(alpha, Sv, Sh, a0, a1, a2, a3, a4, a6, ...
    a7, a5, a8, Fz_r, mu)
persistent C D B E

% init persistent variables: 
if isempty(C)
    C = a0;
    D = mu*(a1*Fz_r^2 + a2*Fz_r);
    B = (a3*sin(a4*atan(Fz_r/a5)))/C/D;
    E = a6*Fz_r^2 + a7*Fz_r + a8;

end
X = alpha+Sh;
phi = (1-E)*X + E/B*atan(B*X);
F_y0 = -(D*sin(C*atan(B*phi)) +Sv);

== matlab function vehicle_model10DOF_2023b/Vehicle/Subsystem/Subsystem4/Tyre Model RR/Combined force ==
  data: F_x0 input; F output; s input; F_y0 input; alpha input; Fx output; Fy output
 function [F, Fx, Fy] = fcn(F_x0, s, F_y0, alpha)


% normalization of s
s = s/100;
alpha_rad = alpha/180*pi;

beta = atan2(sin(alpha_rad), s);

Fx = F_x0*abs(cos(beta));

Fy = F_y0*abs(sin(beta));

F =  F_x0*cos(beta)^2 + F_y0*sin(beta)^2;

== matlab function vehicle_model10DOF_2023b/Vehicle/Subsystem/Subsystem4/Tyre Model RR/brake force  ==
  data: s input; F_x0 output; b0 parameter; b1 parameter; b2 parameter; b3 parameter; b4 parameter; b6 parameter; b7 parameter; b5 parameter; b8 parameter; Fz_f parameter; mu parameter
function F_x0 = fcn(s, b0, b1, b2, b3, b4, b6, b7, b5, b8, Fz_f, mu)
persistent C D B E

% init persistent variables: 
if isempty(C)
    C = b0;
    D = mu*(b1*Fz_f^2 + b2*Fz_f);
    B = (b3*Fz_f^2 + b4*Fz_f)/(C*D)*exp(-b5*Fz_f);
    E = b6*Fz_f^2 + b7*Fz_f + b8;

end
X = s;
phi = (1-E)*X + E/B*atan(B*X);
F_x0 = (D*sin(C*atan(B*phi)));

== matlab function vehicle_model10DOF_2023b/Vehicle/Subsystem/Subsystem4/Tyre Model RR/side force ==
  data: alpha input; Sv input; Sh input; F_y0 output; a0 parameter; a1 parameter; a2 parameter; a3 parameter; a4 parameter; a6 parameter; a7 parameter; a5 parameter; a8 parameter; Fz_r parameter; mu parameter
function F_y0 = fcn(alpha, Sv, Sh, a0, a1, a2, a3, a4, a6, ...
    a7, a5, a8, Fz_r, mu)
persistent C D B E

% init persistent variables: 
if isempty(C)
    C = a0;
    D = mu*(a1*Fz_r^2 + a2*Fz_r);
    B = (a3*sin(a4*atan(Fz_r/a5)))/C/D;
    E = a6*Fz_r^2 + a7*Fz_r + a8;

end
X = alpha+Sh;
phi = (1-E)*X + E/B*atan(B*X);
F_y0 = -(D*sin(C*atan(B*phi)) +Sv);

== matlab function vehicle_model10DOF_2023b/Vehicle/Subsystem1/slip angle [deg] ==
  data: vl_fl input; vc_fl input; vl_fr input; alpha_fl output; vc_fr input; vl_rl input; vc_rl input; alpha_fr output; alpha_rl output; alpha_rr output; vl_rr input; vc_rr input
function [alpha_fl, alpha_fr, alpha_rl, alpha_rr] = slip_angle(vl_fl, ...
    vc_fl, vl_fr, vc_fr, ...
    vl_rl, vc_rl, vl_rr, vc_rr)

alpha_fl = atan2(vl_fl, vc_fl)/pi*180;
alpha_fr = atan2(vl_fr, vc_fr)/pi*180;
alpha_rl = atan2(vl_rl, vc_rl)/pi*180;
alpha_rr = atan2(vl_rr, vc_rr)/pi*180;

== matlab function vehicle_model10DOF_2023b/Vehicle/Subsystem2/vehicle_model10DOF/Wheels ==
  data: Fl_fl input; wfldot output; Fl_fr input; Fl_rl input; Fl_rr input; Tbfl input; Tbfr input; Tbrl input; Tbrr input; wfl input; wfr input; wrl input; wrr input; wfrdot output; wrldot output; wrrdot output; Bd parameter; r parameter; Idf parameter; Idr parameter
function [wfldot, wfrdot, wrldot, wrrdot] = wheels(Fl_fl, Fl_fr, Fl_rl, ...
    Fl_rr, Tbfl, Tbfr, Tbrl, Tbrr, wfl, wfr, wrl, wrr, Bd, r, Idf, Idr)

wfldot = 1/Idf*(-Fl_fl*r - Tbfl - Bd*wfl);
wfrdot = 1/Idf*(-Fl_fr*r - Tbfr - Bd*wfr);
wrldot = 1/Idr*(-Fl_rl*r - Tbrl - Bd*wrl);
wrrdot = 1/Idr*(-Fl_rr*r - Tbrr - Bd*wrr);

== matlab function vehicle_model10DOF_2023b/Vehicle/Subsystem2/vehicle_model10DOF/vehicle6DOF ==
  data: ydotdot output; ydot input; xdotdot output; xdot input; psidot input; psi input; Fx_fl input; Fy_fl input; Fx_fr input; Fy_fr input; Fx_rl input; Fy_rl input; Fx_rr input; Fy_rr input; Fw input; Mw input; psidotdot output; Xdot output; Ydot output; a parameter; b parameter; c parameter; I parameter; m parameter
function [ydotdot, xdotdot, psidotdot, Xdot, Ydot] = dof_6(ydot, xdot, ...
    psidot, psi, Fx_fl, Fy_fl, Fx_fr,  Fy_fr, Fx_rl, Fy_rl, Fx_rr, Fy_rr, ...
    Fw, Mw, a, b, c, I, m)

xdotdot = psidot*ydot + 1/m*(Fx_fl + Fx_fr + Fx_rl + Fx_rr);
ydotdot = -psidot*xdot + 1/m*(Fw + Fy_fl + Fy_fr + Fy_rl+ Fy_rr);
psidotdot = 1/I*(a*(Fy_fl + Fy_fr) - b*(Fy_rl + Fy_rr) + ...
    c*(-Fx_fl + Fx_fr - Fx_rl + Fx_rr) + Mw);
Xdot = xdot*cos(psi) - ydot*sin(psi);
Ydot = xdot*sin(psi) + ydot*cos(psi);

== matlab function vehicle_model10DOF_2023b/wind ==
  data: vw input; Fw output; Mw output; a parameter; b parameter
function [Fw, Mw] = wind(vw, a, b)

Fw = 2.5*pi/2*vw^2;
Mw = (2.5*pi/2 - 3.3*(pi/2)^3)*vw^2 + (a-b)/2*Fw;

== matlab function vehicle_model10DOF_2023b/Vehicle/Subsystem2/vehicle_model10DOF/Subsystem/MATLAB Function ==
  data: Fl input; Fx output; Fc input; delta input; Fy output
function [Fx, Fy] = fcn(Fl, Fc, delta)
Fx = Fl*sin(delta) + Fc*cos(delta);
Fy = Fl*cos(delta) - Fc*sin(delta);

== matlab function vehicle_model10DOF_2023b/Vehicle/Subsystem2/vehicle_model10DOF/Subsystem/MATLAB Function1 ==
  data: Fl input; Fx output; Fc input; delta input; Fy output
function [Fx, Fy] = fcn(Fl, Fc, delta)
Fx = Fl*sin(delta) + Fc*cos(delta);
Fy = Fl*cos(delta) - Fc*sin(delta);

== matlab function vehicle_model10DOF_2023b/Vehicle/Subsystem/Subsystem4/Tyre Model FL/side force ==
  data: alpha input; Sv input; Sh input; F_y0 output; a0 parameter; a1 parameter; a2 parameter; a3 parameter; a4 parameter; a6 parameter; a7 parameter; a5 parameter; a8 parameter; Fz_r parameter; mu parameter
function F_y0 = fcn(alpha, Sv, Sh, a0, a1, a2, a3, a4, a6, ...
    a7, a5, a8, Fz_r, mu)
persistent C D B E

% init persistent variables: 
if isempty(C)
    C = a0;
    D = mu*(a1*Fz_r^2 + a2*Fz_r);
    B = (a3*sin(a4*atan(Fz_r/a5)))/C/D;
    E = a6*Fz_r^2 + a7*Fz_r + a8;

end
X = alpha+Sh;
phi = (1-E)*X + E/B*atan(B*X);
F_y0 = -(D*sin(C*atan(B*phi)) +Sv);

== matlab function vehicle_model10DOF_2023b/Vehicle/Subsystem2/vehicle_model10DOF/Subsystem/MATLAB Function2 ==
  data: Fl input; Fx output; Fc input; delta input; Fy output
function [Fx, Fy] = fcn(Fl, Fc, delta)
Fx = Fl*sin(delta) + Fc*cos(delta);
Fy = Fl*cos(delta) - Fc*sin(delta);

== matlab function vehicle_model10DOF_2023b/Vehicle/Subsystem2/vehicle_model10DOF/Subsystem/MATLAB Function3 ==
  data: Fl input; Fx output; Fc input; delta input; Fy output
function [Fx, Fy] = fcn(Fl, Fc, delta)
Fx = Fl*sin(delta) + Fc*cos(delta);
Fy = Fl*cos(delta) - Fc*sin(delta);

== matlab function vehicle_model10DOF_2023b/Vehicle/Subsystem1/slip ratio [%]/MATLAB Function ==
  data: Tb input; s output; vl input; w input; r parameter
function s = slip_percent(Tb, vl, w, r)

% if breaking Tb > 0
if Tb > 0
    if w == 0 && vl == 0
        s = r-1;
    elseif vl == 0
        s = 1*sign(w);
    else
        s = r*w/vl - 1;
    end
% if driving Tb == 0
else
    if w == 0 && vl == 0
        s = 1-1/r;
    elseif w == 0
        s = -1*sign(vl);
    else
        s = 1 - vl/r/w;
    end
end
% conersion to %
s = s*100;
   


end

== matlab function vehicle_model10DOF_2023b/Vehicle/Subsystem1/MATLAB Function1 ==
  data: x_dot input; vl_fl output; vc_fl output; y_dot input; psi_dot input; delta_f input; delta_r input; vl_fr output; vc_fr output; vl_rl output; vc_rl output; vl_rr output; vc_rr output; a parameter; b parameter; c parameter
function [vl_fl, vc_fl, vl_fr, vc_fr, ...
    vl_rl, vc_rl, vl_rr, vc_rr] = wheel_speeds(x_dot, y_dot, psi_dot, ...
    delta_f, delta_r, a, b, c)

vy_fl = y_dot + a*psi_dot;
vx_fl = x_dot - c*psi_dot;

vy_fr = y_dot + a*psi_dot;
vx_fr = x_dot + c*psi_dot;

vy_rl = y_dot - b*psi_dot;
vx_rl = x_dot - c*psi_dot;

vy_rr = y_dot - b*psi_dot;
vx_rr = x_dot + c*psi_dot;

% Front wheen speeds
vl_fl = vy_fl*sin(delta_f) + vx_fl*cos(delta_f);
vc_fl = vy_fl*cos(delta_f) - vx_fl*sin(delta_f);

vl_fr = vy_fr*sin(delta_f) + vx_fr*cos(delta_f);
vc_fr = vy_fl*cos(delta_f) - vx_fl*sin(delta_f);

%Rear wheel speeds
vl_rl = vy_rl*sin(delta_r) + vx_rl*cos(delta_r);
vc_rl = vy_rl*cos(delta_r) - vx_rl*sin(delta_r);

vl_rr = vy_rr*sin(delta_r) + vx_rr*cos(delta_r);
vc_rr = vy_rr*cos(delta_r) - vx_rr*sin(delta_r);
end

== matlab function vehicle_model10DOF_2023b/Vehicle/Subsystem1/slip ratio [%]/MATLAB Function2 ==
  data: Tb input; s output; vl input; w input; r parameter
function s = slip_percent(Tb, vl, w, r)

% if breaking Tb > 0
if Tb > 0
    if w == 0 && vl == 0
        s = r-1;
    elseif vl == 0
        s = 1*sign(w);
    else
        s = r*w/vl - 1;
    end
% if driving Tb == 0
else
    if w == 0 && vl == 0
        s = 1-1/r;
    elseif w == 0
        s = -1*sign(vl);
    else
        s = 1 - vl/r/w;
    end
end
% conersion to %
s = s*100;
   


end

== matlab function vehicle_model10DOF_2023b/Vehicle/Subsystem1/slip ratio [%]/MATLAB Function3 ==
  data: Tb input; s output; vl input; w input; r parameter
function s = slip_percent(Tb, vl, w, r)

% if breaking Tb > 0
if Tb > 0
    if w == 0 && vl == 0
        s = r-1;
    elseif vl == 0
        s = 1*sign(w);
    else
        s = r*w/vl - 1;
    end
% if driving Tb == 0
else
    if w == 0 && vl == 0
        s = 1-1/r;
    elseif w == 0
        s = -1*sign(vl);
    else
        s = 1 - vl/r/w;
    end
end
% conersion to %
s = s*100;
   


end

== matlab function vehicle_model10DOF_2023b/Vehicle/Subsystem1/slip ratio [%]/MATLAB Function4 ==
  data: Tb input; s output; vl input; w input; r parameter
function s = slip_percent(Tb, vl, w, r)

% if breaking Tb > 0
if Tb > 0
    if w == 0 && vl == 0
        s = r-1;
    elseif vl == 0
        s = 1*sign(w);
    else
        s = r*w/vl - 1;
    end
% if driving Tb == 0
else
    if w == 0 && vl == 0
        s = 1-1/r;
    elseif w == 0
        s = -1*sign(vl);
    else
        s = 1 - vl/r/w;
    end
end
% conersion to %
s = s*100;
   


end

== matlab function vehicle_model10DOF_2023b/internal MPC/BrakingLogic/MATLAB Function ==
  data: delta input; alpha_f input; alpha_r input; M input; Tbfl output; Tbfr output; Tbrl output; Tbrr output; a parameter; b parameter; c parameter; r parameter
function [Tbfl, Tbfr, Tbrl, Tbrr] = braking_logic(delta, alpha_f, alpha_r, M, a, b, c, r)

if (M == 0)
    Tbfl = 0; Tbfr = 0; Tbrl = 0; Tbrr = 0;
else
    if (M >0) % braking the left side
        if (alpha_f - alpha_r >0) %  understeering
            Tbfl = 0; Tbfr = 0; Tbrl = abs(M)*r/(sin(atan(c/b)*sqrt(b^2+c^2))); Tbrr = 0;
        else % oversteering
            Tbfl = abs(M)*r/(sin(atan(c/a) - delta)*sqrt(a^2+c^2)); Tbfr = 0; Tbrl = 0; Tbrr = 0;
        end
    else % braking the right side
        if (alpha_f - alpha_r >0) %  understeering
            Tbfl = 0; Tbfr = 0; Tbrl = 0; Tbrr = abs(M)*r/(sin(atan(c/b)*sqrt(b^2+c^2)));
        else % oversteering 
            Tbfl = 0; Tbfr = abs(M)*r/(sin(atan(c/a) - delta)*sqrt(a^2+c^2)); Tbrl = 0; Tbrr = 0;
        end
    end
end

== matlab function vehicle_model10DOF_2023b/internal MPC/BrakingLogic/MATLAB Function1 ==
  data: alpha_fl input; alpha_f output; alpha_r output; alpha_fr input; alpha_rl input; alpha_rr input
function [alpha_f, alpha_r] = alpha_xy_2_alpha_x(alpha_fl, alpha_fr, ...
    alpha_rl, alpha_rr)

alpha_f = 0.5*alpha_fl + 0.5*alpha_fr;
alpha_r = 0.5*alpha_rl + 0.5*alpha_rr;

== matlab function vehicle_model10DOF_2023b/internal MPC/simplified internal MPC/Subsystem/MATLAB Function ==
  data: Q input; M output; Delta output
function [M, Delta] = MPC(Q)
if Q  ~= 1 
    Delta = 0;
    M = 0;
else
end

== matlab function vehicle_model10DOF_2023b/internal MPC/full internal MPC1/Subsystem/MATLAB Function ==
  data: Q input; M output; Delta output
function [M, Delta] = MPC(Q)
if Q  ~= 1 
    Delta = 0;
    M = 0;
else
end

== matlab function vehicle_model10DOF_2023b/Trajectory replaner/Trajectory MPC/MATLAB Function ==
  data: u input; y output
function y = fcn(u)

y = u;

== matlab function vehicle_model10DOF_2023b/Vehicle/Subsystem/Subsystem4/Tyre Model FL/brake force  ==
  data: s input; F_x0 output; b0 parameter; b1 parameter; b2 parameter; b3 parameter; b4 parameter; b6 parameter; b7 parameter; b5 parameter; b8 parameter; Fz_f parameter; mu parameter
function F_x0 = fcn(s, b0, b1, b2, b3, b4, b6, b7, b5, b8, Fz_f, mu)
persistent C D B E

% init persistent variables: 
if isempty(C)
    C = b0;
    D = mu*(b1*Fz_f^2 + b2*Fz_f);
    B = (b3*Fz_f^2 + b4*Fz_f)/(C*D)*exp(-b5*Fz_f);
    E = b6*Fz_f^2 + b7*Fz_f + b8;

end
X = s;
phi = (1-E)*X + E/B*atan(B*X);
F_x0 = (D*sin(C*atan(B*phi)));

== matlab function vehicle_model10DOF_2023b/Vehicle/Subsystem/Subsystem4/Tyre Model FL/Combined force ==
  data: F_x0 input; F output; s input; F_y0 input; alpha input; Fx output; Fy output
 function [F, Fx, Fy] = fcn(F_x0, s, F_y0, alpha)


% normalization of s
s = s/100;
alpha_rad = alpha/180*pi;

beta = atan2(sin(alpha_rad), s);

Fx = F_x0*abs(cos(beta));

Fy = F_y0*abs(sin(beta));

F =  F_x0*cos(beta)^2 + F_y0*sin(beta)^2;

== matlab function vehicle_model10DOF_2023b/Vehicle/Subsystem/Subsystem4/Tyre Model FR/Combined force ==
  data: F_x0 input; F output; s input; F_y0 input; alpha input; Fx output; Fy output
 function [F, Fx, Fy] = fcn(F_x0, s, F_y0, alpha)


% normalization of s
s = s/100;
alpha_rad = alpha/180*pi;

beta = atan2(sin(alpha_rad), s);

Fx = F_x0*abs(cos(beta));

Fy = F_y0*abs(sin(beta));

F =  F_x0*cos(beta)^2 + F_y0*sin(beta)^2;

== matlab function vehicle_model10DOF_2023b/Vehicle/Subsystem/Subsystem4/Tyre Model FR/brake force  ==
  data: s input; F_x0 output; b0 parameter; b1 parameter; b2 parameter; b3 parameter; b4 parameter; b6 parameter; b7 parameter; b5 parameter; b8 parameter; Fz_f parameter; mu parameter
function F_x0 = fcn(s, b0, b1, b2, b3, b4, b6, b7, b5, b8, Fz_f, mu)
persistent C D B E

% init persistent variables: 
if isempty(C)
    C = b0;
    D = mu*(b1*Fz_f^2 + b2*Fz_f);
    B = (b3*Fz_f^2 + b4*Fz_f)/(C*D)*exp(-b5*Fz_f);
    E = b6*Fz_f^2 + b7*Fz_f + b8;

end
X = s;
phi = (1-E)*X + E/B*atan(B*X);
F_x0 = (D*sin(C*atan(B*phi)));
